simulink model "motorcycle_simulink"  (R2021a)
settings: Solver=VariableStepAuto  StartTime=0.0  StopTime=10.0  RelTol=1e-3
settings Model: Creator=martina.elle  LastModifiedBy=avall

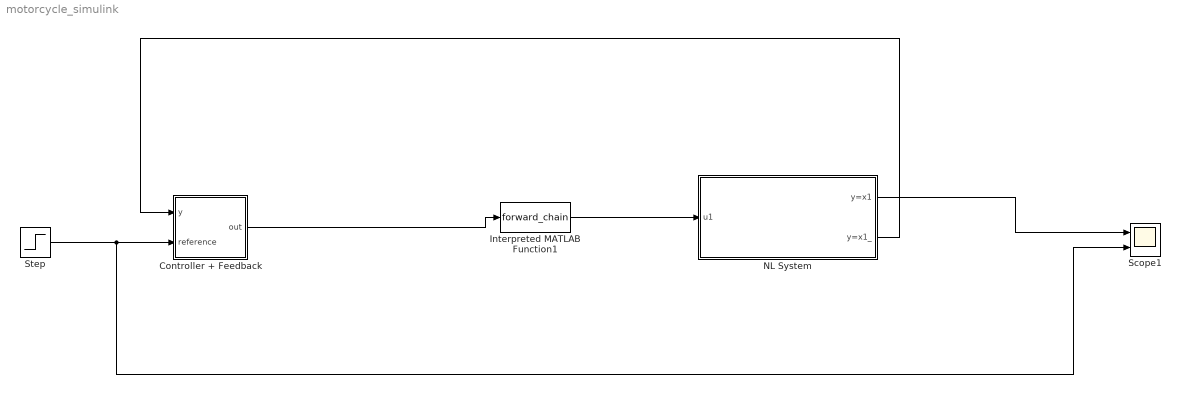
== system motorcycle_simulink ==
  Controller + Feedback : Subsystem
  Interpreted MATLAB Function1 : MATLABFcn  MATLABFcn=forward_chain  OutputDimensions=1
  NL System : Subsystem
  Scope1 : Scope  NumInputPorts=2
  Step : Step  Time=0  After=30  SampleTime=0
  wires:
  Controller + Feedback/1(out) -> Interpreted MATLAB Function1/1
  Step/1 -> Scope1/2, Controller + Feedback/2(reference)
  Interpreted MATLAB Function1/1 -> NL System/1(u1)
  NL System/2(y=x1_) -> Controller + Feedback/1(y)
  NL System/1(y=x1) -> Scope1/1

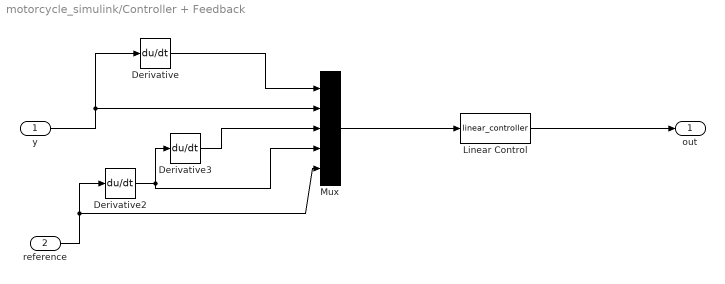
== system motorcycle_simulink/Controller + Feedback ==
  y : Inport
  reference : Inport  Port=2
  Derivative : Derivative
  Derivative2 : Derivative
  Derivative3 : Derivative
  Linear Control : MATLABFcn  MATLABFcn=linear_controller  OutputDimensions=2
  Mux : Mux  Inputs=5
  out : Outport
  wires:
  y/1 -> Derivative/1, Mux/2
  reference/1 -> Mux/5, Derivative2/1
  Derivative2/1 -> Mux/4, Derivative3/1
  Derivative/1 -> Mux/1
  Derivative3/1 -> Mux/3
  Mux/1 -> Linear Control/1
  Linear Control/1 -> out/1

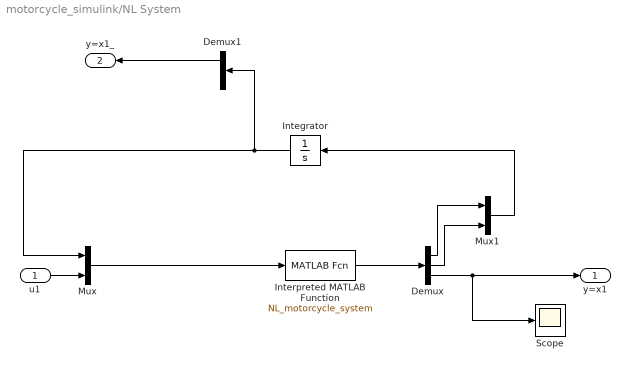
== system motorcycle_simulink/NL System ==
  u1 : Inport
  Demux : Demux  Outputs=3
  Demux1 : Demux  Outputs=2
  Integrator : Integrator  InitialCondition=[10 10]
  Interpreted MATLAB Function : MATLABFcn  MATLABFcn=NL_motorcycle_system  OutputDimensions=3
  Mux : Mux  Inputs=2
  Mux1 : Mux  Inputs=2
  Scope : Scope
  y=x1 : Outport
  y=x1_ : Outport  Port=2
  wires:
  u1/1 -> Mux/2
  Demux/2 -> Mux1/2
  Mux/1 -> Interpreted MATLAB Function/1
  Mux1/1 -> Integrator/1
  Integrator/1 -> Demux1/1, Mux/1
  Demux/1 -> Mux1/1
  Interpreted MATLAB Function/1 -> Demux/1
  Demux/3 -> Scope/1, y=x1/1
  Demux1/1 -> y=x1_/1
